simulink model "atrias_gear_dynamics"  (R2017a)
settings: Solver=ode45  StartTime=0.0  StopTime=sim_t  RelTol=1e-3  EnableMultiTasking=on
values from neighbouring files (symbols this model uses):
  N = grid_slice*1000    [createGrid.m]
  nm = fn_set_vnmc_params(sm, sample_time)    [kernel_scores_NM_mismatch.m]    (also in main_ATRIAS_cluster.m)
  nmc_BLCtrlPar = nmc.BLCtrlPar    [kernel_scores_NM_mismatch.m]    (also in main_ATRIAS_cluster.m)
  nmc_FPCtrlPar = nmc.FPCtrlPar    [kernel_scores_NM_mismatch.m]    (also in main_ATRIAS_cluster.m)
  nmc_LLCtrlPar = nmc.LLCtrlPar    [kernel_scores_NM_mismatch.m]    (also in main_ATRIAS_cluster.m)
  nmc_StCtrlPar = nmc.StCtrlPar    [kernel_scores_NM_mismatch.m]    (also in main_ATRIAS_cluster.m)
  nmc_SwCtrlPar = nmc.SwCtrlPar    [kernel_scores_NM_mismatch.m]    (also in main_ATRIAS_cluster.m)
  nmc_TrCtrlPar = nmc.TrCtrlPar    [kernel_scores_NM_mismatch.m]    (also in main_ATRIAS_cluster.m)
  nStep_switchCtrl = 10    [main_ATRIAS_cluster.m]
  nStep_thr = 1000    [createSimInitial.m]    (also in main_ATRIAS_cluster.m)
  rc_CtrlPar = [rc.k_placement, rc.T_step, rc.Cd, rc.kpt, rc.kdt, rc.desired_theta, rc.desired_z, rc.kpz, rc.kdz]    [kernel_scores_NM_mismatch.m]    (also in main_ATRIAS_cluster.m)
  sm = fn_set_MechParams(sm)    [kernel_scores_NM_mismatch.m]    (also in main_ATRIAS_cluster.m = fn_set_MechParams(sm,perturb))
  test_VNMC = 1    [createSimInitial.m]    (also in main_ATRIAS_cluster.m = 0)
undefined symbols (not defined in the file or in its folder): delta_phi_max, delta_phi_max_buffer, delta_phi_min, DiscIntNeverNeededParam, Discrete, idc, initial_dx_estimate, initial_dy_estimate, initial_dz_estimate, initial_z_estimate, kd_shin_max, kd_shin_min, kd_splay_max, kd_splay_min, kd_thigh_max, kd_thigh_min, kp_shin_max, kp_shin_min, kp_splay_max, kp_splay_min, kp_thigh_max, kp_thigh_min, mc, min_splay_angle, min_splay_buffer, phi_shin_max, phi_shin_max_buffer, phi_shin_min, phi_shin_min_buffer, phi_thigh_max, phi_thigh_max_buffer, phi_thigh_min, phi_thigh_min_buffer, rad, rc, s, sample_time, sgn, sim_d, t_friction, Time, X, Y, Z
libraries: sm_lib x206, nesl_utility x132, simulink x77, simulink_extras x24, mblibv1 x4, ctrlSharedLib x4, commnoisgen2 x1, dspswit3 x1
(part 2 of 17)

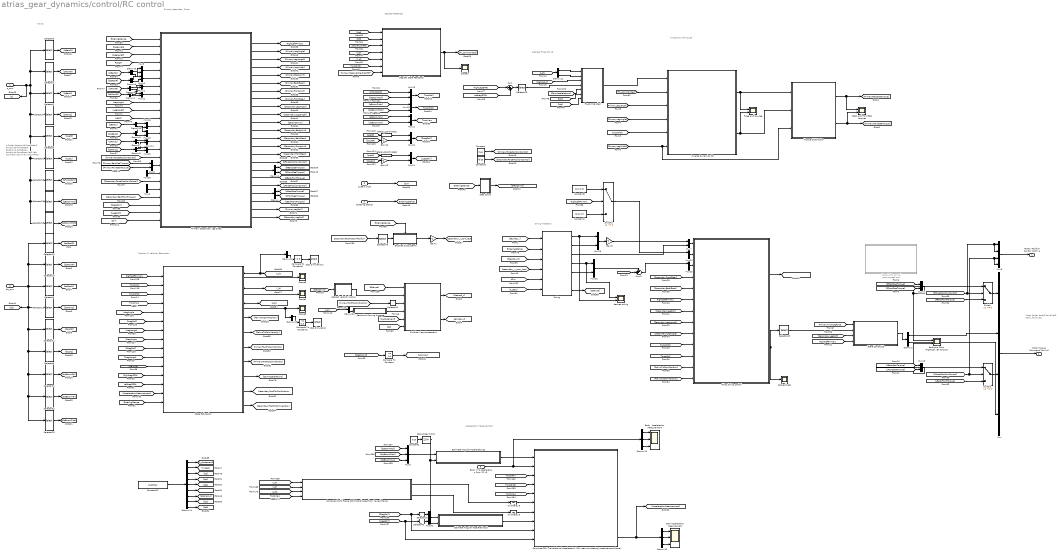
== system atrias_gear_dynamics/control/RC control ==
  note: Motor Order:
      |
      | backR
      | frontR
      | latR
      | backL
      | frontL
      | latL
  note: Inverse Dynamics 2D
  note: Desired Fz sent to ID
  note: Primary/secondary Swap
  note: Sagittal Feedback
  note: Swing Trajectory
  note: Inputs
  note: q Order:
      |
      | backJointR
      | backGearR
      | frontJointR
      | frontGearR
      |
      | backJointL
      | backGearL
      | frontJointL
      | frontGearL
      |
      | latR
      | latL
      |
      | boomRoll
      | boomYaw
      | boomPitch
  note: Position & Velocity Estimation
  note: Acceleration Measurement
  q_cmu : Inport
  dq_cmu : Inport  Port=2
  system clock : Inport  Port=3
  Entering Stance : Inport  Port=4
  Body XYZ Acceleration [m/s^2] x3 : Inport  Port=5
  Atrias Swing control : Subsystem
  Back and Front Right/Left SEA torques : Scope  NumInputPorts=2
  Back and Front SEA torques : Scope  NumInputPorts=2
  Body  Acceleration Measurement : Scope  NumInputPorts=3
  COM Acceleration Measurement : Scope  NumInputPorts=3
  Compare To Constant : simulink/Logic and Bit Operations/Compare To Constant  relop=>=  const=1.0  OutDataTypeStr=boolean
  Compare To Constant1 : simulink/Logic and Bit Operations/Compare To Constant  relop=<=  const=0.3  OutDataTypeStr=boolean
  Compare To Constant2 : simulink/Logic and Bit Operations/Compare To Constant  relop=>=  const=5  OutDataTypeStr=boolean
  Compute COM Translational Acceleration (IMU uses non-rotating measurement frame) : MATLAB Function  TreatAsAtomicUnit=on
  Compute World Frame COM Coordinates from Yawed Frame : MATLAB Function  TreatAsAtomicUnit=on
  Constant : Constant  Value=true
  Constant1 : Constant  Value=false
  Constant12 : Constant  Value=rc_CtrlPar
  Constant2 : Constant  Value=true
  Constant4 : Constant  Value=[0.12 0]
  Constant8 : Constant  Value=[-0.12 0]
  Demux{,1..11,15..16,21} (15 alike) : Demux  Outputs=2
  Demux12 : Demux  Outputs=3
  Demux13 : Demux  Outputs=3
  Demux14 : Demux  Outputs=9
  Enabled Subsystem1 : Subsystem  TreatAsAtomicUnit=on
  Estimate Angular Accelerations2 : Subsystem
  Estimate Angular Accelerations3 : Subsystem
  F_leg and tau_leg : Scope  NumInputPorts=2
  Fz_commanded : Subsystem
  Gain{1,5,12..13} (4 alike) : Gain  Gain=-1
  Inverse Dynamics 2D : Subsystem
  Mux : Mux
  Mux{6..26,28,30,32} (24 alike) : Mux  Inputs=2
  Mux3 : Mux
  Mux5 : Mux  Inputs=3
  Primary Secondary Leg Swap : Subsystem
  Recursive Moving Average : Subsystem
  Sagittal State Feedback : MATLAB Function  TreatAsAtomicUnit=on
  Scope{1,3..5} (4 alike) : Scope
  Selector1 : Selector  InputPortWidth=13  IndexOptions=Index vector (dialog)  Indices=[10]  OutputSizes=1
  Selector10 : Selector  InputPortWidth=13  IndexOptions=Index vector (dialog)  Indices=[7 8]  OutputSizes=1
  Selector11 : Selector  InputPortWidth=13  IndexOptions=Index vector (dialog)  Indices=[9]  OutputSizes=1
  Selector12 : Selector  InputPortWidth=13  IndexOptions=Index vector (dialog)  Indices=[1 2]  OutputSizes=1
  Selector13 : Selector  InputPortWidth=13  IndexOptions=Index vector (dialog)  Indices=[3 4]  OutputSizes=1
  Selector15 : Selector  InputPortWidth=2  IndexOptions=Index vector (dialog)  Indices=[2]  OutputSizes=1
  Selector16 : Selector  InputPortWidth=2  IndexOptions=Index vector (dialog)  Indices=[2]  OutputSizes=1
  Selector18 : Selector  InputPortWidth=13  IndexOptions=Index vector (dialog)  Indices=[13]  OutputSizes=1
  Selector2 : Selector  InputPortWidth=13  IndexOptions=Index vector (dialog)  Indices=[5 6]  OutputSizes=1
  Selector20 : Selector  InputPortWidth=13  IndexOptions=Index vector (dialog)  Indices=[13]  OutputSizes=1
  Selector21 : Selector  InputPortWidth=13  IndexOptions=Index vector (dialog)  Indices=[11]  OutputSizes=1
  Selector22 : Selector  InputPortWidth=13  IndexOptions=Index vector (dialog)  Indices=[12]  OutputSizes=1
  Selector23 : Selector  InputPortWidth=13  IndexOptions=Index vector (dialog)  Indices=[11]  OutputSizes=1
  Selector28 : Selector  InputPortWidth=13  IndexOptions=Index vector (dialog)  Indices=[12]  OutputSizes=1
  Selector4 : Selector  InputPortWidth=13  IndexOptions=Index vector (dialog)  Indices=[7 8]  OutputSizes=1
  Selector40 : Selector  InputPortWidth=3  IndexOptions=Index vector (dialog)  Indices=[1 2]  OutputSizes=1
  Selector41 : Selector  InputPortWidth=3  IndexOptions=Index vector (dialog)  Indices=1  OutputSizes=1
  Selector42 : Selector  InputPortWidth=2  IndexOptions=Index vector (dialog)  Indices=[2]  OutputSizes=1
  Selector43 : Selector  InputPortWidth=3  IndexOptions=Index vector (dialog)  Indices=[1]  OutputSizes=1
  Selector5 : Selector  InputPortWidth=13  IndexOptions=Index vector (dialog)  Indices=[9]  OutputSizes=1
  Selector6 : Selector  InputPortWidth=13  IndexOptions=Index vector (dialog)  Indices=[1 2]  OutputSizes=1
  Selector7 : Selector  InputPortWidth=13  IndexOptions=Index vector (dialog)  Indices=[3 4]  OutputSizes=1
  Selector8 : Selector  InputPortWidth=13  IndexOptions=Index vector (dialog)  Indices=[10]  OutputSizes=1
  Selector9 : Selector  InputPortWidth=13  IndexOptions=Index vector (dialog)  Indices=[5 6]  OutputSizes=1
  Simbicon leg placcement : Subsystem
  State Estimation : Subsystem
  Step Count : Subsystem
  Stop Simulation : Stop
  Stop Simulation1 : Stop
  Sum : Sum  Inputs=|++
  Sum2 : Sum  Inputs=-+|
  Swing : Subsystem
  Switch : Switch  Criteria=u2 ~= 0
  Switch1 : Switch  Criteria=u2 ~= 0
  Switch2 : Switch  Criteria=u2 ~= 0
  Torque Distribution : Subsystem
  Unit Delay5 : UnitDelay  SampleTime=sample_time
  Unit Delay6 : UnitDelay  SampleTime=sample_time
  Zero-Order Hold1 : ZeroOrderHold  SampleTime=sample_time
  desired beta : Scope
  desired swing : Scope  NumInputPorts=2
  desired velocity lookup : MATLAB Function  TreatAsAtomicUnit=on
  lateralControl2D : Subsystem
  lateral_PID_control : Subsystem  Commented=on
  lateral_coordinates : Fcn  Expr=pi/2-u
  lateral_coordinates1 : Fcn  Expr=pi/2-u
  Force / Position Control [1/0] x4 : Outport  OutputWhenDisabled=reset  InitialOutput=[0 0 0 0 0 0]
  Motor Torque Command [Nm] x6 : Outport  Port=2  OutputWhenDisabled=reset  InitialOutput=[0 0 0 0 0 0]
  tag scope: EnteringStance=global, PrimaryFootToComPosition=global, RightLeftPrimary=global, SecondaryFootToComPosition=global, TorsoPitch=global, TorsoRoll=global, TorsoYaw=global, X_dX=global, Y_dY=global, Z_dZ=global, desired_xd=global, tSim=global
  wires:
  ? -> Mux20/2
  [LLegRoll] -> State Estimation/6(Left Leg Roll [rad rad/s])
  Selector9/1 -> [dqBackL]
  ? -> Mux6/2
  ? -> Mux26/2
  ? -> Mux6/1
  desired velocity lookup/1(desired_xd) -> Simbicon leg placcement/2(dx_des [m/s])
  State Estimation/7(Primary Foot to COM Velocity [m/s m/s m/s]) -> [PrimaryFootToComVelocity]
  State Estimation/6(Primary Foot to COM Position [m m m]) -> [PrimaryFootToComPosition]
  State Estimation/1("Horizontal COM [m, m/s]") -> Scope3/1, Demux16/1, [X_dX]
  Selector1/1 -> [qLatL]
  Selector2/1 -> [qBackL]
  ? -> Mux26/1
  Selector7/1 -> [qFrontR]
  Selector6/1 -> [qBackR]
  ? -> Mux25/2
  Selector12/1 -> [dqBackR]
  Selector11/1 -> [dqLatR]
  Selector8/1 -> [dqLatL]
  Selector22/1 -> [dqBoomYaw]
  [RLegLength] -> State Estimation/10(Right Leg Length [m m/s])
  [LLegAngle] -> State Estimation/5(Left Leg Sagittal Angle [rad rad/s])
  [TorsoPitch] -> State Estimation/3(Torso Pitch [rad rad/s])
  dq_cmu/1 -> Selector9/1, Selector13/1, Selector12/1, [dq], Selector10/1, Selector11/1, Selector8/1, Selector21/1, Selector22/1, Selector20/1
  Selector13/1 -> [dqFrontR]
  State Estimation/10(Secondary to COM Velocity [m/s m/s m/s]) -> [SecondaryFootToComVelocity]
  Selector21/1 -> [dqBoomRoll]
  Selector20/1 -> [dqBoomPitch]
  [RLegRoll] -> State Estimation/9(Right Leg Roll [rad rad/s])
  Selector23/1 -> [qTorsoRoll]
  Selector18/1 -> [qBoomPitch]
  [TorsoRoll] -> State Estimation/2(Torso Roll [rad rad/s])
  Selector28/1 -> [qBoomYaw]
  Selector4/1 -> [qFrontL]
  q_cmu/1 -> [q], Selector1/1, Selector23/1, Selector28/1, Selector18/1, Selector5/1, Selector4/1, Selector2/1, Selector7/1, Selector6/1
  Selector10/1 -> [dqFrontL]
  Demux21/2 -> Recursive Moving Average/1(dx [m/s])
  Gain1/1 -> [secondary_x_com_last]
  State Estimation/4(Pelvis to COM Position [m m m]) -> [PelvisToComPosition]
  [LLegLength] -> State Estimation/7(Left Leg Length [m m/s])
  State Estimation/9(Secondary to COM Position [m m m]) -> [SecondaryFootToComPosition]
  [tStance] -> Simbicon leg placcement/1(Ts [s])
  Selector5/1 -> [qLatR]
  Entering Stance/1 -> [EnteringStance]
  [desired_x] -> Swing/1(desired_x)
  Simbicon leg placcement/1(desired_footsstep) -> [desired_x]
  [TorsoYaw] -> State Estimation/4(Torso Yaw [rad rad/s])
  [PrimaryFootToComPosition] -> Selector41/1
  [X_dX] -> Demux21/1
  [PrimaryLegLength] -> Inverse Dynamics 2D/3(Leg Length [m m/s])  "Primary Leg Length [position, velocity]"
  [PrimaryLegAngle] -> Inverse Dynamics 2D/4(Leg Angle [rad rad/s])  "Primary Leg Angle  [position, velocity]"
  [TorsoPitch] -> Inverse Dynamics 2D/5(Torso Pitch [rad rad/s])  "Torso Pitch [position, velocity]"
  [PrimaryLegWidth] -> Inverse Dynamics 2D/6(Primary w [m]), Torque Distribution/3(Primary Leg Width [m])
  Inverse Dynamics 2D/1(Leg Force [N]) -> F_leg and tau_leg/1, Torque Distribution/1(Leg Force [N])  "Virtual Leg Force to Command"
  Inverse Dynamics 2D/2(Leg Torque [Nm]) -> F_leg and tau_leg/2, Torque Distribution/2(Leg Torque [Nm])  "Virtual Leg Torque to Command"
  Torque Distribution/1(Back Torque [Nm]) -> Back and Front SEA torques/1, [PrimaryBackSeaTorque]
  Torque Distribution/2(Front Torque [Nm]) -> Back and Front SEA torques/2, [PrimaryFrontSeaTorque]
  [SecondaryBackFrontTorque] -> Primary Secondary Leg Swap/21(Secondary Back/Front Motor Torque [Nm Nm])
  Mux26/1 -> Primary Secondary Leg Swap/18(Primary Back/Front Motor Torque [Nm Nm])
  [SecondaryForcePositionControl] -> Primary Secondary Leg Swap/19(Secondary Force/Position Control [1/0])
  [PrimaryForcePositionControl] -> Primary Secondary Leg Swap/16(Primary Force/Position Control [1/0])
  Demux9/2 -> Mux13/2
  Demux9/1 -> Mux16/2
  Demux10/2 -> Mux13/1
  Demux10/1 -> Mux16/1
  [qBackL] -> Demux10/1
  [dqBackL] -> Demux9/1
  Demux8/2 -> Mux15/2
  Demux8/1 -> Mux14/2
  Demux7/2 -> Mux15/1
  Demux7/1 -> Mux14/1
  Mux15/1 -> Primary Secondary Leg Swap/15(L Front Gear [rad rad/s])
  Mux14/1 -> Primary Secondary Leg Swap/14(L Front Joint [rad rad/s])
  Mux13/1 -> Primary Secondary Leg Swap/13(L Back Gear [rad rad/s])
  Mux16/1 -> Primary Secondary Leg Swap/12(L Back Joint [rad rad/s])
  [dqFrontL] -> Demux8/1
  [qFrontL] -> Demux7/1
  Demux5/2 -> Mux10/2
  Demux5/1 -> Mux9/2
  Demux6/2 -> Mux10/1
  Demux6/1 -> Mux9/1
  [qBackR] -> Demux6/1
  [dqBackR] -> Demux5/1
  Demux4/2 -> Mux12/2
  Demux4/1 -> Mux11/2
  Demux3/2 -> Mux12/1
  Demux3/1 -> Mux11/1
  Mux12/1 -> Primary Secondary Leg Swap/8(R Front Gear [rad rad/s])
  Mux11/1 -> Primary Secondary Leg Swap/7(R Front Joint [rad rad/s])
  Mux10/1 -> Primary Secondary Leg Swap/6(R Back Gear [rad rad/s])
  Mux9/1 -> Primary Secondary Leg Swap/5(R Back Joint [rad rad/s])
  [dqFrontR] -> Demux4/1
  [qFrontR] -> Demux3/1
  [PrimaryBackSeaTorque] -> Mux8/1
  [PrimaryFrontSeaTorque] -> Mux8/2
  Mux8/1 -> Primary Secondary Leg Swap/17(Primary Back/Front SEA Torque [Nm Nm])
  Mux6/1 -> Primary Secondary Leg Swap/20(Secondary Back/Front SEA Torque [Nm Nm])
  [LLegW] -> Primary Secondary Leg Swap/11(L Leg w [m])
  [LLegLength] -> Primary Secondary Leg Swap/10(L Leg Length [m m/s])
  [LLegAngle] -> Primary Secondary Leg Swap/9(L Leg Angle [rad rad/s])
  [RLegW] -> Primary Secondary Leg Swap/4(R Leg w [m])
  [RLegLength] -> Primary Secondary Leg Swap/3(R Leg Length [m m/s])
  [RLegAngle] -> Primary Secondary Leg Swap/2(R Leg Angle [rad rad/s])
  [RLegRoll] -> Primary Secondary Leg Swap/22("Right Leg Roll [rad, rad/s]")
  [LLegRoll] -> Primary Secondary Leg Swap/23("Left Leg Roll [rad, rad/s]")
  Primary Secondary Leg Swap/1(Right/Left Primary [1/0]) -> [RightLeftPrimary]
  Primary Secondary Leg Swap/21(L Back/Front Motor Torque [Nm Nm]) -> [LBackFrontTorque]
  Primary Secondary Leg Swap/18(R Back/Front Motor Torque [Nm Nm]) -> [RBackFrontTorque]
  Primary Secondary Leg Swap/16(R Force/Position Control [1/0]) -> [RForcePositionControl]
  Primary Secondary Leg Swap/19(L Force/Position Control [1/0]) -> [LForcePositionControl]
  Primary Secondary Leg Swap/11(Secondary Leg w [m]) -> [SecondaryW]
  Primary Secondary Leg Swap/15(Secondary Front Gear [rad rad/s]) -> [SecondaryFrontGear]
  Primary Secondary Leg Swap/14(Secondary Front Joint [rad rad/s]) -> [SecondaryFrontJoint]
  Primary Secondary Leg Swap/13(Secondary Back Gear [rad rad/s]) -> [SecondaryBackGear]
  Primary Secondary Leg Swap/12(Secondary Back Joint [rad rad/s]) -> [SecondaryBackJoint]
  Primary Secondary Leg Swap/8(Primary Front Gear [rad rad/s]) -> [PrimaryFrontGear]
  Primary Secondary Leg Swap/7(Primary Front Joint [rad rad/s]) -> [PrimaryFrontJoint]
  Primary Secondary Leg Swap/6(Primary Back Gear [rad rad/s]) -> [PrimaryBackGear]
  Primary Secondary Leg Swap/5(Primary Back Joint [rad rad/s]) -> [PrimaryBackJoint]
  Demux1/2 -> [RFrontSeaTorque]
  Demux1/1 -> [RBackSeaTorque]
  Primary Secondary Leg Swap/17(R Back/Front SEA Torque [Nm Nm]) -> Demux1/1
  Demux/2 -> [LFrontSeaTorque]
  Demux/1 -> [LBackSeaTorque]
  Primary Secondary Leg Swap/20(L Back/Front SEA Torque [Nm Nm]) -> Demux/1
  Primary Secondary Leg Swap/9(Secondary Leg Angle [rad rad/s]) -> [SecondaryLegAngle]
  Primary Secondary Leg Swap/10(Secondary Leg Length [rad rad/s]) -> [SecondaryLegLength]
  Primary Secondary Leg Swap/3(Primary Leg Length [m m/s]) -> [PrimaryLegLength]
  Primary Secondary Leg Swap/4(Primary Leg w [m]) -> [PrimaryLegWidth]
  Primary Secondary Leg Swap/2(Primary Leg Angle [rad rad/s]) -> [PrimaryLegAngle]
  Primary Secondary Leg Swap/22("Primary Leg Roll [rad, rad/s]") -> [PrimaryLegRoll]
  Primary Secondary Leg Swap/23("Secondary Leg Roll [rad, rad/s]") -> [SecondaryLegRoll]
  Switch1/1 -> Mux/3
  [LBackFrontTorque] -> Switch1/3
  [RBackFrontTorque] -> Switch/3
  Demux2/1 -> Mux/2
  Switch/1 -> Mux/1
  [LForcePositionControl] -> Switch1/2, Mux3/3, Mux3/4
  [RForcePositionControl] -> Switch/2, Mux3/1, Mux3/2
  Mux3/1 -> Force / Position Control [1/0] x4/1
  Mux/1 -> Motor Torque Command [Nm] x6/1
  Demux2/2 -> Mux/4
  [RBackSeaTorque] -> Mux17/1
  [RFrontSeaTorque] -> Mux17/2
  Mux17/1 -> Switch/1, Back and Front Right/Left SEA torques/1
  [LBackSeaTorque] -> Mux18/1
  [LFrontSeaTorque] -> Mux18/2
  Mux18/1 -> Back and Front Right/Left SEA torques/2, Switch1/1
  Constant/1 -> [PrimaryForcePositionControl]
  Constant1/1 -> [SecondaryForcePositionControl]
  [SecondaryFrontGear] -> Atrias Swing control/4(Secondary Front Gear [rad rad/s])
  [SecondaryBackGear] -> Atrias Swing control/5(Secondary Back Gear [rad rad/s])
  [dqBoomYaw] -> Mux21/2
  [qBoomYaw] -> Mux21/1
  [qBoomPitch] -> Mux19/1
  Gain12/1 -> Mux22/2
  Gain13/1 -> Mux24/2
  lateral_coordinates1/1 -> Mux24/1
  lateral_coordinates/1 -> Mux22/1
  Mux24/1 -> [LLegRoll]
  Mux22/1 -> [RLegRoll]
  [dqLatL] -> Gain13/1
  [qLatL] -> lateral_coordinates1/1
  [dqLatR] -> Gain12/1
  [qLatR] -> lateral_coordinates/1
  [dqBoomPitch] -> Mux19/2
  Mux19/1 -> [TorsoPitch]
  Mux23/1 -> [TorsoRoll]
  Mux21/1 -> [TorsoYaw]
  [dqBoomRoll] -> Mux23/2
  [qTorsoRoll] -> Mux23/1
  Atrias Swing control/1(Back Front Motor Torques [Nm Nm]) -> [SecondaryBackFrontTorque]
  Atrias Swing control/2(Desired Swing Beta [rad rad/s]) -> Selector40/1, desired beta/1
  [RightLeftPrimary] -> Atrias Swing control/6(Right or Left Stance [1 or 0])
  [SecondaryLegRoll] -> Atrias Swing control/7(Secondary Leg Roll [rad rad/s])
  [TorsoRoll] -> Atrias Swing control/11(Torso Roll [rad rad/s])
  [TorsoPitch] -> Atrias Swing control/10(Torso Pitch [rad rad/s])
  [SecondaryLegAngle] -> Atrias Swing control/9(Secondary Leg Angle [rad rad/s])
  [SecondaryLegLength] -> Atrias Swing control/8(Secondary Leg Length [m m/s])
  Sum2/1 -> Mux25/1
  [Z_dZ] -> Sum2/2
  Mux20/1 -> Atrias Swing control/2(Y COM  from Secondary Foot Desired [m m/s m/s^2])
  Mux25/1 -> Atrias Swing control/3(Z COM  from Secondary Foot Desired [m m/s m/s^2])
  [RightLeftPrimary] -> lateralControl2D/4(RightLeftPrimary [1 or 0])
  [Z_dZ] -> Demux11/1
  Demux11/1 -> Fz_commanded/1(measured_z)
  [TorsoPitch] -> Sagittal State Feedback/6(theta_dtheta)
  [Z_dZ] -> Sagittal State Feedback/5(z_dz)
  Mux7/1 -> Atrias Swing control/1(X COM from Secondary Foot Desired [m m/s m/s^2])
  Mux32/1 -> Sum2/1
  [PelvisToComPosition] -> Atrias Swing control/12(Pelvis to COM Position [m] x3)
  [PelvisToComVelocity] -> Atrias Swing control/13(Pelvis to COM Velocity [m/s] x3)
  [EnteringStance] -> Primary Secondary Leg Swap/1(Entering Stance [1/0])
  [RightLeftPrimary] -> Switch2/2
  Switch2/1 -> Mux20/1
  Constant8/1 -> Switch2/1
  Constant4/1 -> Switch2/3
  [X_dX] -> Sagittal State Feedback/4(x_dx)
  [tSim] -> Primary Secondary Leg Swap/24(System Time [s])
  [EnteringStance] -> Step Count/1(In1)
  Step Count/1(Out1) -> [StepCount]
  [PrimaryMeasuredVerticalGRF] -> Sagittal State Feedback/7(GRF_z)
  Demux11/2 -> Fz_commanded/2(measured_zd)
  Fz_commanded/1(Fz_commanded) -> Inverse Dynamics 2D/1(Desired Vertical GRF [N])
  Sagittal State Feedback/1(Fx) -> [Fx_commanded], Scope1/1
  [Fx_commanded] -> Inverse Dynamics 2D/2(Desired Forward GRF [N])
  [EnteringStance] -> Swing/2(EnteringStance)
  [StepCount] -> Swing/3(nstep)
  [tSim] -> Swing/5(tSim)
  Swing/2(xd) -> Mux28/2
  Swing/5(zd) -> Mux32/2
  Swing/7(tStance_last) -> [tStance]
  Swing/1(x) -> desired swing/2, Mux28/1
  Swing/4(z) -> desired swing/1, Mux32/1
  lateralControl2D/1(Lateral Torque command [R L]) -> Demux2/1
  Swing/3(xdd) -> Mux7/2
  [secondary_x_com_last] -> Swing/4(secondary_x)
  Mux28/1 -> Gain5/1
  Gain5/1 -> Mux7/1
  Enabled Subsystem1/1(Out1) -> Gain1/1
  [EnteringStance] -> Enabled Subsystem1/Enable
  [SecondaryFootToComPosition] -> Selector43/1
  Selector43/1 -> Enabled Subsystem1/1(In1)
  Selector41/1 -> Simbicon leg placcement/3(Foot2CoM)
  system clock/1 -> [tSim]
  State Estimation/2("Lateral COM [m, m/s]") -> Scope4/1, [Y_dY]
  State Estimation/5(Pelvis to COM Velocity [m/s m/s m/s]) -> [PelvisToComVelocity]
  [RightLeftPrimary] -> State Estimation/1(Right or Left [1/0])
  Recursive Moving Average/1(dx_avg [m/s]) -> Simbicon leg placcement/4(dx_avg [m/s])
  [RLegAngle] -> State Estimation/8(Right Leg Sagittal Angle [rad rad/s])
  [RightLegGRFs] -> State Estimation/12(Right GRF [X Z] [N N])
  [LeftLegGRFs] -> State Estimation/13(Left GRF [X Z] [N N])
  [EnteringStance] -> State Estimation/15(Entering Stance [1/0])
  [AccelerationMeasurement] -> State Estimation/14(" Acceleration Measurement [m/s^2] x3")
  [TorsoYaw] -> Compute World Frame COM Coordinates from Yawed Frame/4(torso_yaw)
  [Z_dZ] -> Compute World Frame COM Coordinates from Yawed Frame/3(Z_dZ)
  [Y_dY] -> Compute World Frame COM Coordinates from Yawed Frame/2(Y_dY)
  [X_dX] -> Compute World Frame COM Coordinates from Yawed Frame/1(X_dX)
  Compute World Frame COM Coordinates from Yawed Frame/1(com_position_world) -> Unit Delay5/1
  Compute World Frame COM Coordinates from Yawed Frame/2(com_velocity_world) -> Unit Delay6/1
  Unit Delay6/1 -> Compute COM Translational Acceleration (IMU uses non-rotating measurement frame)/7(com_velocity_world)
  Unit Delay5/1 -> Compute COM Translational Acceleration (IMU uses non-rotating measurement frame)/6(com_position_world)
  [TorsoYaw] -> Compute COM Translational Acceleration (IMU uses non-rotating measurement frame)/5(torso_yaw)
  Estimate Angular Accelerations3/1(Angular Accelerations [rad/s^2] x2) -> Compute COM Translational Acceleration (IMU uses non-rotating measurement frame)/8(hip_roll_accelerations)
  Estimate Angular Accelerations2/1(Angular Accelerations [rad/s^2] x3) -> Compute COM Translational Acceleration (IMU uses non-rotating measurement frame)/1(torso_angular_accelerations)
  Zero-Order Hold1/1 -> Estimate Angular Accelerations3/2(Enabled), Estimate Angular Accelerations2/2(Enabled)
  Mux5/1 -> Estimate Angular Accelerations2/1(Angular Velocities [rad/s] x3)
  [TorsoRoll] -> Compute COM Translational Acceleration (IMU uses non-rotating measurement frame)/3(torso_roll)
  [TorsoPitch] -> Compute COM Translational Acceleration (IMU uses non-rotating measurement frame)/4(torso_pitch)
  Demux12/3 -> COM Acceleration Measurement/3
  Demux12/1 -> COM Acceleration Measurement/1
  Demux12/2 -> COM Acceleration Measurement/2
  Compute COM Translational Acceleration (IMU uses non-rotating measurement frame)/6(com_acceleration_yawed) -> [AccelerationMeasurement], Demux12/1
  [dqBoomRoll] -> Mux5/1
  [dqBoomPitch] -> Mux5/2
  [dqBoomYaw] -> Mux5/3
  Mux30/1 -> Estimate Angular Accelerations3/1(Angular Velocities [rad/s] x2)
  Selector42/1 -> Mux30/2
  Selector16/1 -> Mux30/1
  [LLegRoll] -> Compute COM Translational Acceleration (IMU uses non-rotating measurement frame)/10(left_hip_roll), Selector42/1
  [RLegRoll] -> Compute COM Translational Acceleration (IMU uses non-rotating measurement frame)/9(right_hip_roll), Selector16/1
  [walking] -> State Estimation/11(Enable Kalman Filtering [1/0])
  [StepCount] -> Compare To Constant/1
  Compare To Constant/1 -> [walking]
  Constant2/1 -> Zero-Order Hold1/1
  State Estimation/8(COM Acceleration [m/s^2] x3) -> [ComAccelerations]
  [ComAccelerations] -> Fz_commanded/5(COM XYZ Acceleration [m/s^2] x3)
  [SecondaryLegRoll] -> lateralControl2D/3(SecondaryLegRoll)
  Selector40/1 -> lateralControl2D/2(desired_SecondaryLegRoll)
  [PrimaryAxialLegForce] -> lateralControl2D/1(Primary Axial Leg Force [N])
  Demux13/3 -> Body  Acceleration Measurement/3
  Demux13/1 -> Body  Acceleration Measurement/1
  Demux13/2 -> Body  Acceleration Measurement/2
  Body XYZ Acceleration [m/s^2] x3/1 -> Demux13/1, Compute COM Translational Acceleration (IMU uses non-rotating measurement frame)/2(imu_translational_accelerations_body)
  [k_placement] -> Simbicon leg placcement/5(k_placement)
  [T_step] -> Swing/6(T_step)
  [Cd] -> Simbicon leg placcement/6(Cd)
  [kpt] -> Sagittal State Feedback/1(kpt)
  [kdt] -> Sagittal State Feedback/2(kdt)
  Selector15/1 -> Fz_commanded/4("Primary Measured Vertical [N}")
  State Estimation/3("Vertical COM [m, m/s]") -> Demux15/1, Scope5/1, [Z_dZ]
  Compare To Constant1/1 -> Stop Simulation/1
  Demux15/1 -> Compare To Constant1/1
  Compare To Constant2/1 -> Stop Simulation1/1
  Demux16/2 -> Compare To Constant2/1
  [StepCount] -> desired velocity lookup/1(nStep)
  [RightLegGRFs] -> Sum/1
  [LeftLegGRFs] -> Sum/2
  Sum/1 -> Selector15/1
  Simbicon leg placcement/2(desired_speed) -> [desired_xd]
  [desired_theta] -> Sagittal State Feedback/3(desired_theta)
  [desired_z] -> Fz_commanded/3(desired_z)
  [kpz] -> Fz_commanded/6(kpz)
  [kdz] -> Fz_commanded/7(kdz)
  Demux14/9 -> [kdz]
  Demux14/2 -> [T_step]
  Demux14/5 -> [kdt]
  Demux14/4 -> [kpt]
  Constant12/1 -> Demux14/1
  Demux14/6 -> [desired_theta]
  Demux14/8 -> [kpz]
  Demux14/7 -> [desired_z]
  Demux14/3 -> [Cd]
  Demux14/1 -> [k_placement]

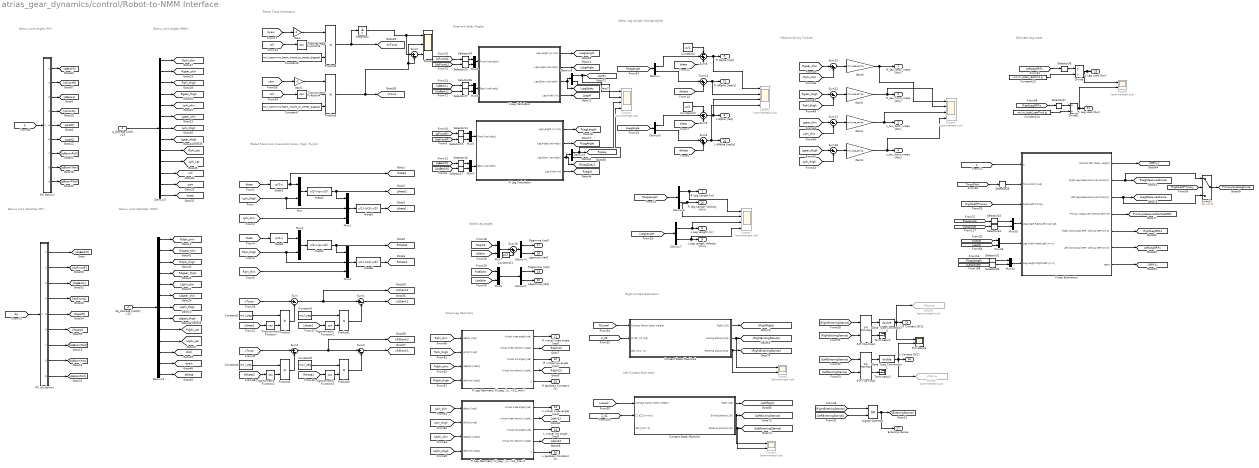
== system atrias_gear_dynamics/control/Robot-to-NMM Interface ==
  note: Global Robot Link Kinematics
      | (torso, thigh, fb_link)
  note: Planar Torso Kinematics
  note: Alpha, Leg Length
      | (change alpha)
  note: Demux Joint
      | Angles (NMC)
  note: Demux Joint
      | Velocities (NMC)
  note: Knee and Splay Angles
  note: Virtual Leg Geometry
  note: Measure Spring Torques
  note: Estimate Leg Loads
  note: Global Leg Angles
  note: Demux Joint
      | Angles (RC)
  note: Demux Joint
      | Velocities (RC)
  note: Left Contact Estimation
  note: Right Contact Estimation
  q_discrete [rad] x13 : Inport
  dq_discrete [rad/2] x13 : Inport  Port=2
  Constant1 : Constant  Value=pi/2
  Constant11 : Constant  Value=pi/2
  Constant12 : Constant  Value=pi/2
  Constant13 : Constant  Value=mc.m_total_real*mc.g
  Constant14 : Constant  Value=mc.m_total_real*mc.g
  Constant{2..5} (4 alike) : Constant  Value=mc.l_seg
  Constant6 : Constant  Value=mc.l_boom+mc.boom_mount_to_center_diagonal
  Constant7 : Constant  Value=mc.l_boom+mc.boom_mount_to_center_diagonal
  Contact State Machine : Subsystem
  Contact State Machine1 : Subsystem
  Data Type Conversion1 : DataTypeConversion  OutDataTypeStr=double
  Data Type Conversion3 : DataTypeConversion  OutDataTypeStr=double
  Demux{,1,4..9} (8 alike) : Demux  Outputs=2
  Demux2 : Demux  Outputs=13
  Demux3 : Demux  Outputs=13
  Divide : Product  Inputs=*/
  Divide1 : Product  Inputs=*/
  Force Estimation : Subsystem
  Gain : Gain  Gain=-1
  Gain1 : Gain  Gain=-1
  Gain{3..6} (4 alike) : Gain  Gain=mc.k_leg_spring
  Goto81 : Goto  Commented=on  GotoTag=RStance  TagVisibility=global
  Goto84 : Goto  Commented=on  GotoTag=LStance  TagVisibility=global
  Integrator : Integrator
  L Leg Calculator : Subsystem
  Logical Operator : Logic  Operator=OR  AllPortsSameDT=off  OutDataTypeStr=boolean
  Mux{,2,4..9,33..35} (11 alike) : Mux  Inputs=2
  Mux1 : Mux  Inputs=3
  Mux3 : Mux  Inputs=3
  Product{,1..3} (4 alike) : Product
  Product4 : Product  Inputs=3
  Product5 : Product  Inputs=3
  R Leg Calculator : Subsystem
  "R Leg Geometry f(l_seg, l_v, v12_max)" : Subsystem
  "R Leg Geometry f(l_seg, l_v, v12_max)1" : Subsystem
  R/L Stance : Scope  NumInputPorts=2
  RC Demux : Subsystem
  RC dq demux : Subsystem
  S-R Flip-Flop1 : simulink_extras/Flip Flops/S-R Flip-Flop  initial_condition=0
  S-R Flip-Flop2 : simulink_extras/Flip Flops/S-R Flip-Flop  initial_condition=0
  Scope : Scope  NumInputPorts=3
  Scope2 : Scope  Commented=on  NumInputPorts=2
  Scope3 : Scope  Commented=on  NumInputPorts=2
  Scope{4..7} (4 alike) : Scope  Commented=on  NumInputPorts=4
  Scope8 : Scope  Commented=on  NumInputPorts=2
  Selector{14..17,24..27,31..35} (13 alike) : Selector  InputPortWidth=2  IndexOptions=Index vector (dialog)  Indices=[1]  OutputSizes=1
  Selector36 : Selector  InputPortWidth=2  IndexOptions=Index vector (dialog)  Indices=[2]  OutputSizes=1
  Selector37 : Selector  InputPortWidth=2  IndexOptions=Index vector (dialog)  Indices=[2]  OutputSizes=1
  Sum{,1..3,7,10..13} (9 alike) : Sum  Inputs=|+-
  Sum14 : Sum  Inputs=|++
  Sum18 : Sum  Inputs=|++
  Sum4 : Sum  Inputs=|++
  Sum5 : Sum  Inputs=-++
  Sum6 : Sum  Inputs=-++
  Switch1 : Switch  Criteria=u2 ~= 0
  Terminator1 : Terminator
  Terminator2 : Terminator
  Trigonometric Function{,1..4,6} (6 alike) : Trigonometry  Operator=cos
  theta1 : Fcn  Expr=u(1)+(pi-u(2))
  theta2 : Fcn  Expr=u(1)+(pi-u(2))
  theta3 : Fcn  Expr=pi/2-u
  theta4 : Fcn  Expr=pi/2-u
  theta5 : Fcn  Expr=u(1)-(u(3)-u(2))
  theta6 : Fcn  Expr=u(1)-(u(3)-u(2))
  R_tau_back_meas [Nm] : Outport
  R_tau_front_meas [Nm] : Outport  Port=2
  L_tau_back_meas [Nm] : Outport  Port=3
  L_tau_front_meas [Nm] : Outport  Port=4
  R Alpha [rad] : Outport  Port=5
  L Alpha [rad] : Outport  Port=6
  R Leg Length [m] : Outport  Port=7
  L Leg Length [m] : Outport  Port=8
  L Leg Length Velocity [m/s] : Outport  Port=9
  R Leg Length Velocity [m/s] : Outport  Port=10
  R virtual knee angle [rad] : Outport  Port=11
  R virtual hip angle [rad] : Outport  Port=12
  L virtual knee angle [rad] : Outport  Port=13
  L virtual hip angle [rad] : Outport  Port=14
  R Jacobian Constant (k) : Outport  Port=15
  L Jacobian Constant (k) : Outport  Port=16
  Rgamma [rad] : Outport  Port=17
  Lgamma [rad] : Outport  Port=18
  Rdgamma [rad] : Outport  Port=19
  Ldgamma [rad] : Outport  Port=20
  R dAlpha [rad/s] : Outport  Port=21
  L dAlpha [rad/s] : Outport  Port=22
  L Leg Load [bw] : Outport  Port=23
  R Leg Load [bw] : Outport  Port=24
  R Contact [0/1] : Outport  Port=25
  L Contact [0/1] : Outport  Port=26
  Entering stance : Outport  Port=27
  tag scope: LLegAngle=global, LLegLength=global, LLegMeasuredForce=global, LLegSplay=global, LLegW=global, Ldgear_shin=global, Ldgear_thigh=global, Ldphi12=global, Ldphi23=global, Ldphi_Lat=global, Ldphi_shin=global, Ldphi_thigh=global, LeftLegGRFs=global, Lgear_shin=global, Lgear_thigh=global, Lphi_Lat=global, Lphi_shin=global, Lphi_thigh=global, Lsplay=global, Ltheta1=global, Ltheta2=global, PrimaryAxialLegForce=global, PrimaryMeasuredVerticalGRF=global, RLegAngle=global, RLegLength=global, RLegMeasuredForce=global, RLegW=global, Rdgear_shin=global, Rdgear_thigh=global, Rdphi12=global, Rdphi23=global, Rdphi_Lat=global, Rdphi_shin=global, Rdphi_thigh=global, Rgear_shin=global, Rgear_thigh=global, RightLegGRFs=global, Rphi_Lat=global, Rphi_shin=global, Rphi_thigh=global, Rsplay=global, Rtheta1=global, Rtheta2=global, droll=global, dtheta=global, dxTorso=global, dyaw=global, roll=global, theta3=global, theta=global, xLShank1=global, xLShank2=global, xRShank1=global, xRShank2=global, xTorso=global, yaw=global
  wires:
  Sum3/1 -> [xRShank1]
  Sum2/1 -> [xRShank2], Sum3/1
  Product3/1 -> Sum3/2
  Trigonometric Function3/1 -> Product3/2
  Constant2/1 -> Product/1
  Trigonometric Function/1 -> Product/2
  Sum1/1 -> [xLShank1]
  Constant3/1 -> Product1/1
  Trigonometric Function2/1 -> Product2/2
  Product1/1 -> Sum1/2
  [Rtheta2] -> Trigonometric Function2/1
  Sum/1 -> [xLShank2], Sum1/1
  [Ltheta1] -> Trigonometric Function1/1
  Product/1 -> Sum/2
  Product2/1 -> Sum2/2
  [xTorso] -> Sum2/1
  [Rtheta1] -> Trigonometric Function3/1
  Constant4/1 -> Product2/1
  Constant5/1 -> Product3/1
  [xTorso] -> Sum/1
  [Ltheta2] -> Trigonometric Function/1
  Product4/1 -> [dxTorso], Integrator/1
  Trigonometric Function1/1 -> Product1/2
  [dyaw] -> Gain/1
  [theta] -> theta3/1
  [Lphi_thigh] -> Mux1/2, Mux/2
  theta3/1 -> Mux/1, [theta3]
  Mux/1 -> theta2/1
  theta2/1 -> Mux1/1, [Ltheta2]
  Mux1/1 -> theta5/1
  [Lphi_shin] -> Mux1/3
  [theta] -> theta4/1
  [Rphi_thigh] -> Mux3/2, Mux2/2
  theta4/1 -> Mux2/1
  Mux2/1 -> theta1/1
  theta1/1 -> Mux3/1, [Rtheta2]
  Mux3/1 -> theta6/1
  [Rphi_shin] -> Mux3/3
  theta5/1 -> [Ltheta1]
  theta6/1 -> [Rtheta1]
  [theta] -> Sum6/3
  Constant1/1 -> Sum6/1
  Sum6/1 -> Scope5/1, R Alpha [rad]/1
  Demux3/1 -> [Rphi_shin]
  Demux3/2 -> [Rgear_shin]
  Demux3/3 -> [Rphi_thigh]
  Demux3/4 -> [Rgear_thigh]
  Demux3/5 -> [Lphi_shin]
  Demux3/6 -> [Lgear_shin]
  Demux3/7 -> [Lphi_thigh]
  Demux3/8 -> [Lgear_thigh]
  Demux3/9 -> [Rphi_Lat]
  Demux3/10 -> [Lphi_Lat]
  Demux3/11 -> [roll]
  Demux3/12 -> [yaw]
  Demux3/13 -> [theta]
  Demux2/13 -> [dtheta]
  Demux2/8 -> [Ldgear_thigh]
  Demux2/10 -> [Ldphi_Lat]
  Demux2/6 -> [Ldgear_shin]
  Demux2/9 -> [Rdphi_Lat]
  Demux2/11 -> [droll]
  Demux2/12 -> [dyaw]
  Demux2/4 -> [Rdgear_thigh]
  Demux2/5 -> [Ldphi_shin]
  Demux2/7 -> [Ldphi_thigh]
  Demux2/1 -> [Rdphi_shin]
  Demux2/3 -> [Rdphi_thigh]
  Demux2/2 -> [Rdgear_shin]
  dq_discrete [rad/2] x13/1 -> Demux2/1
  Trigonometric Function6/1 -> Product4/2
  [roll] -> Trigonometric Function6/1
  Constant6/1 -> Product4/3
  [Lgear_shin] -> Sum11/1
  Sum11/1 -> Gain4/1
  [Lphi_shin] -> Sum11/2
  Gain4/1 -> Scope6/3, L_tau_back_meas [Nm]/1
  [Lgear_thigh] -> Sum10/1
  Sum10/1 -> Gain3/1
  [Lphi_thigh] -> Sum10/2
  Gain3/1 -> Scope6/4, L_tau_front_meas [Nm]/1
  [Rgear_shin] -> Sum13/1
  Sum13/1 -> Gain6/1
  [Rphi_shin] -> Sum13/2
  Gain6/1 -> Scope6/1, R_tau_back_meas [Nm]/1
  [Rgear_thigh] -> Sum12/1
  Sum12/1 -> Gain5/1
  [Rphi_thigh] -> Sum12/2
  Gain5/1 -> Scope6/2, R_tau_front_meas [Nm]/1
  Demux6/1 -> Scope7/1, R Leg Length [m]/1
  Demux7/1 -> Scope7/3, L Leg Length [m]/1
  [Rphi_thigh] -> "R Leg Geometry f(l_seg, l_v, v12_max)"/2(qFront [rad])
  [Rphi_shin] -> "R Leg Geometry f(l_seg, l_v, v12_max)"/1(qBack [rad])
  [Rdphi_shin] -> "R Leg Geometry f(l_seg, l_v, v12_max)"/3(dqBack [rad/s])
  [Rdphi_thigh] -> "R Leg Geometry f(l_seg, l_v, v12_max)"/4(dqFront [rad/s])
  "R Leg Geometry f(l_seg, l_v, v12_max)"/4(virtual hip velocity [rad/s]) -> [Rdphi23]
  "R Leg Geometry f(l_seg, l_v, v12_max)"/2(virtual knee velocity [rad/s]) -> [Rdphi12]
  "R Leg Geometry f(l_seg, l_v, v12_max)"/5(k) -> R Jacobian Constant (k)/1
  [Lphi_thigh] -> "R Leg Geometry f(l_seg, l_v, v12_max)1"/2(qFront [rad])
  [Lphi_shin] -> "R Leg Geometry f(l_seg, l_v, v12_max)1"/1(qBack [rad])
  [Ldphi_shin] -> "R Leg Geometry f(l_seg, l_v, v12_max)1"/3(dqBack [rad/s])
  [Ldphi_thigh] -> "R Leg Geometry f(l_seg, l_v, v12_max)1"/4(dqFront [rad/s])
  "R Leg Geometry f(l_seg, l_v, v12_max)1"/5(k) -> L Jacobian Constant (k)/1
  "R Leg Geometry f(l_seg, l_v, v12_max)"/3(virtual hip angle [rad]) -> R virtual hip angle [rad]/1
  "R Leg Geometry f(l_seg, l_v, v12_max)"/1(virtual knee angle [rad]) -> R virtual knee angle [rad]/1
  "R Leg Geometry f(l_seg, l_v, v12_max)1"/1(virtual knee angle [rad]) -> L virtual knee angle [rad]/1
  "R Leg Geometry f(l_seg, l_v, v12_max)1"/3(virtual hip angle [rad]) -> L virtual hip angle [rad]/1
  "R Leg Geometry f(l_seg, l_v, v12_max)1"/2(virtual knee velocity [rad/s]) -> [Ldphi12]
  "R Leg Geometry f(l_seg, l_v, v12_max)1"/4(virtual hip velocity [rad/s]) -> [Ldphi23]
  Constant11/1 -> Sum18/2
  [Ralpha] -> Mux7/1
  [Lalpha] -> Mux7/2
  Mux7/1 -> Sum18/1
  Sum18/1 -> Demux4/1
  Demux4/1 -> Rgamma [rad]/1
  Demux4/2 -> Lgamma [rad]/1
  [Rdalpha] -> Mux6/1
  [Ldalpha] -> Mux6/2
  Mux6/1 -> Demux1/1
  Demux1/1 -> Rdgamma [rad]/1
  Demux1/2 -> Ldgamma [rad]/1
  q_discrete [rad] x13/1 -> Demux3/1
  RC Demux/1(Out1) -> [qBackR]
  RC Demux/2(Out2) -> [qFrontR]
  RC Demux/3(Out3) -> [qBackL]
  RC Demux/4(Out4) -> [qFrontL]
  RC Demux/5(Out5) -> [qLatR]
  RC Demux/6(Out6) -> [qLatL]
  RC Demux/7(Out7) -> [qBoomRoll]
  RC Demux/8(Out8) -> [qBoomYaw]
  RC Demux/9(Out9) -> [qBoomPitch]
  [q] -> RC Demux/1(In1)
  [dq] -> RC dq demux/1(In1)
  RC dq demux/1(Out1) -> [dqBackR]
  RC dq demux/2(Out2) -> [dqFrontR]
  RC dq demux/3(Out3) -> [dqBackL]
  RC dq demux/4(Out4) -> [dqFrontL]
  RC dq demux/5(Out5) -> [dqLatR]
  RC dq demux/6(Out6) -> [dqLatL]
  RC dq demux/7(Out7) -> [dqBoomRoll]
  RC dq demux/8(Out8) -> [dqBoomYaw]
  RC dq demux/9(Out9) -> [dqBoomPitch]
  L Leg Calculator/4(Leg Width [m]) -> [LLegW]
  Selector26/1 -> Mux8/1
  Selector27/1 -> Mux8/2
  Selector25/1 -> Mux9/2
  Selector24/1 -> Mux9/1
  L Leg Calculator/3(Leg Splay [rad rad/s]) -> Demux8/1, [LLegSplay]
  L Leg Calculator/2(Leg Angle [rad rad/s]) -> [LLegAngle]
  L Leg Calculator/1("Leg Length [m m/s] ") -> [LLegLength]
  Mux8/1 -> L Leg Calculator/2(Back [rad rad/s])
  Mux9/1 -> L Leg Calculator/1(Front [rad rad/s])
  [dqFrontL] -> Selector25/1
  [qFrontL] -> Selector24/1
  [dqBackL] -> Selector27/1
  [qBackL] -> Selector26/1
  R Leg Calculator/4(Leg Width [m]) -> [RLegW]
  Selector16/1 -> Mux4/1
  Selector17/1 -> Mux4/2
  Selector15/1 -> Mux5/2
  Selector14/1 -> Mux5/1
  R Leg Calculator/3(Leg Splay [rad rad/s]) -> Demux9/1, [RLegSplay]
  R Leg Calculator/2(Leg Angle [rad rad/s]) -> [RLegAngle]
  [dqFrontR] -> Selector15/1
  [qFrontR] -> Selector14/1
  [dqBackR] -> Selector17/1
  [qBackR] -> Selector16/1
  R Leg Calculator/1("Leg Length [m m/s] ") -> [RLegLength]
  Mux4/1 -> R Leg Calculator/2(Back [rad rad/s])
  Mux5/1 -> R Leg Calculator/1(Front [rad rad/s])
  [RLegAngle] -> Demux/1
  Demux/1 -> Sum6/2
  [dtheta] -> Sum14/2
  Demux/2 -> Sum14/1
  Sum14/1 -> Scope5/2, R dAlpha [rad/s]/1
  [theta] -> Sum5/3
  Constant12/1 -> Sum5/1
  Sum5/1 -> Scope5/3, L Alpha [rad]/1
  [LLegAngle] -> Demux5/1
  Demux5/1 -> Sum5/2
  [dtheta] -> Sum4/2
  Demux5/2 -> Sum4/1
  Sum4/1 -> Scope5/4, L dAlpha [rad/s]/1
  Demux6/2 -> Scope7/2, R Leg Length Velocity [m/s]/1
  [RLegLength] -> Demux6/1
  Demux7/2 -> Scope7/4, L Leg Length Velocity [m/s]/1
  [LLegLength] -> Demux7/1
  [RLegW] -> Mux33/1
  [LLegW] -> Mux33/2
  [RLegLength] -> Selector31/1
  [LLegLength] -> Selector32/1
  Selector31/1 -> Mux34/1
  Selector32/1 -> Mux34/2
  Selector34/1 -> Mux35/2
  [RLegAngle] -> Selector33/1
  [LLegAngle] -> Selector34/1
  Selector33/1 -> Mux35/1
  [TorsoPitch] -> Selector35/1
  [q] -> Force Estimation/1(q)
  Selector35/1 -> Force Estimation/2(Torso Pitch [rad])
  [RightLeftPrimary] -> Force Estimation/3(Right/Left Primary)
  Force Estimation/3(Left Leg Measured Axial Force [N]) -> Switch1/3, [LLegMeasuredForce]
  Force Estimation/2(Right Leg Measured Axial Force [N]) -> Switch1/1, [RLegMeasuredForce]
  Mux35/1 -> Force Estimation/4(Leg Angle Right/Left [rad rad])
  Mux33/1 -> Force Estimation/5(Leg Width Right/Left [m m])
  Mux34/1 -> Force Estimation/6(Leg Length Right/Left [m m])
  Force Estimation/5("Right [horizontal GRF, vertical GRF] [N N]") -> [RightLegGRFs]
  Force Estimation/6("Left [horizontal GRF, vertical GRF] [N N]") -> [LeftLegGRFs]
  Force Estimation/7(GRFx) -> [GRFx]
  Force Estimation/4(Primary Measured Vertical GRF [N]) -> [PrimaryMeasuredVerticalGRF]
  Force Estimation/1(Vertical GRF [body weight]) -> [GRFy]
  Constant13/1 -> Divide/2
  Selector36/1 -> Divide/1
  [LeftLegGRFs] -> Selector36/1
  Divide/1 -> Scope8/1, L Leg Load [bw]/1
  Constant14/1 -> Divide1/2
  Selector37/1 -> Divide1/1
  [RightLegGRFs] -> Selector37/1
  Divide1/1 -> Scope8/2, R Leg Load [bw]/1
  [Z_dZ] -> Contact State Machine/2("[Z dZ] [m m/s]")
  Contact State Machine/2(Exiting Stance [1/0]) -> Scope3/1, [LeftExitingStance]
  Contact State Machine/1(flight [1/0]) -> [Leftflight]
  [Z_dZ] -> Contact State Machine1/2("[Z dZ] [m m/s]")
  Contact State Machine1/1(flight [1/0]) -> [Rightflight]
  [RLLoad] -> Contact State Machine1/1(Contact Factor [body weight])
  [LLLoad] -> Contact State Machine/1(Contact Factor [body weight])
  Contact State Machine/3(Entering stance [1/0]) -> Scope3/2, [LeftEnteringStance]
  Demux8/1 -> Scope4/1, [Lsplay]
  Demux9/1 -> Scope4/3, [Rsplay]
  Data Type Conversion3/1 -> Goto81/1, R/L Stance/1, R Contact [0/1]/1
  [RightEnteringStance] -> Logical Operator/1
  [LeftEnteringStance] -> Logical Operator/2
  Logical Operator/1 -> Entering stance/1, [EnteringStance]
  [RightEnteringStance] -> S-R Flip-Flop1/1
  [RightExitingStance] -> S-R Flip-Flop1/2
  S-R Flip-Flop1/1 -> Data Type Conversion3/1
  S-R Flip-Flop1/2 -> Terminator1/1
  Data Type Conversion1/1 -> Goto84/1, R/L Stance/2, L Contact [0/1]/1
  [LeftEnteringStance] -> S-R Flip-Flop2/1
  [LeftExitingStance] -> S-R Flip-Flop2/2
  S-R Flip-Flop2/1 -> Data Type Conversion1/1
  S-R Flip-Flop2/2 -> Terminator2/1
  [yaw] -> Gain1/1
  Trigonometric Function4/1 -> Product5/2
  [roll] -> Trigonometric Function4/1
  Constant7/1 -> Product5/3
  Product5/1 -> Sum7/2, Scope/2, [xTorso]
  Integrator/1 -> Sum7/1, Scope/1
  Sum7/1 -> Scope/3
  Contact State Machine1/2(Exiting Stance [1/0]) -> Scope2/1, [RightExitingStance]
  Contact State Machine1/3(Entering stance [1/0]) -> Scope2/2, [RightEnteringStance]
  Demux8/2 -> Scope4/2
  Demux9/2 -> Scope4/4
  [RightLeftPrimary] -> Switch1/2
  Switch1/1 -> [PrimaryAxialLegForce]
  Gain/1 -> Product4/1
  Gain1/1 -> Product5/1

== system atrias_gear_dynamics/control/Virtual Neuromuscular Control ==
  note: High-Level
      | Control
  note: Neural
      | Control
  note: Muscle
      | Dynamics
  note: Jacobian Mapping
  Constant10 : Constant  Value=nmc_TrCtrlPar
  Constant12 : Constant  Value=nmc_BLCtrlPar
  Constant2 : Constant  Value=nmc_LLCtrlPar
  Constant5 : Constant  Value=nmc_StCtrlPar
  Constant6 : Constant  Value=nmc_FPCtrlPar
  Constant9 : Constant  Value=nmc_SwCtrlPar
  Higher Control Layer : Subsystem
  Muscle Layer : Subsystem
  Neural Control Layer : Subsystem
  Torque Distribution : Subsystem
  RtauB_des [Nm] : Outport
  RtauF_des [Nm] : Outport  Port=2
  LtauB_des [Nm] : Outport  Port=3
  LtauF_des [Nm] : Outport  Port=4
  tag scope: FPCtrlPar=global, Jinv_trans_L=global, Jinv_trans_R=global, LLCtrlPar=global, StCtrlPar=global, SwCtrlPar=global, TrCtrlPar=global, theta0=global
  wires:
  Torque Distribution/6(L J_inv_transpose [2x2]) -> [Jinv_trans_L]
  Torque Distribution/5(L tauF [Nm]) -> LtauF_des [Nm]/1
  Torque Distribution/4(L tauB [Nm]) -> LtauB_des [Nm]/1
  Torque Distribution/3(R J_inv_transpose [2x2]) -> [Jinv_trans_R]
  [LM12] -> Torque Distribution/4(L tauK_des [Nm])
  [LM23] -> Torque Distribution/5(L tauH_des [Nm])
  [k_R] -> Torque Distribution/3(R Jacobian Constant (k))
  [k_L] -> Torque Distribution/6(L Jacobian Constant (k))
  Torque Distribution/1(R tauB [Nm]) -> RtauB_des [Nm]/1
  Torque Distribution/2(R tauF [Nm]) -> RtauF_des [Nm]/1
  [RM23] -> Torque Distribution/2(R tauH_des [Nm])
  [RM12] -> Torque Distribution/1(R tauK_des [Nm])
  Constant6/1 -> [FPCtrlPar]
  Constant10/1 -> [TrCtrlPar]
  Constant9/1 -> [SwCtrlPar]
  Constant2/1 -> [LLCtrlPar]
  Constant5/1 -> [StCtrlPar]
  Constant12/1 -> [theta0]

== system atrias_gear_dynamics/control/switch Ctrl ==
  VNMC : Inport
  RC : Inport  Port=2
  Constant : Constant  Value=0
  Demux1 : Demux  Outputs=2
  Demux2 : Demux  Outputs=2
  Mux7 : Mux  Inputs=2
  Scope : Scope  Commented=on  NumInputPorts=5
  Scope1 : Scope  NumInputPorts=5
  Switch{1..4} (4 alike) : Switch  Criteria=u2 > Threshold  Threshold=.5
  selected : Outport
  wires:
  Switch2/1 -> Scope/4, selected/1
  Switch1/1 -> Switch2/1
  Constant/1 -> Switch1/2
  [RFootCnt] -> Scope1/1, Switch3/2
  VNMC/1 -> Demux1/1, [vnmc_trq]
  RC/1 -> Demux2/1, [rc_trq]
  Demux1/1 -> Scope1/3, Switch3/1
  Demux2/1 -> Scope1/5, Switch3/3
  [LFootCnt] -> Scope1/2, Switch4/2
  Demux1/2 -> Switch4/1
  Demux2/2 -> Switch4/3
  Switch3/1 -> Scope1/4, Mux7/1
  Switch4/1 -> Mux7/2
  Mux7/1 -> [hybrid_trq]
  [rc_trq] -> Scope/3, Switch2/3
  [vnmc_on] -> Scope/5, Switch2/2
  [vnmc_trq] -> Scope/1, Switch1/3
  [hybrid_trq] -> Scope/2, Switch1/1

== system atrias_gear_dynamics/ATRIAS_sim/Discrete Derivative/discrete difference ==
  note: q Order:
      |
      | backJointR
      | backGearR
      | frontJointR
      | frontGearR
      |
      | backJointL
      | backGearL
      | frontJointL
      | frontGearL
      |
      | latR
      | latL
      |
      | boomRoll
      | boomYaw
      | boomPitch
  in : Inport
  Demux : Demux  Outputs=13
  Mux : Mux  Inputs=13
  difference : simulink/Discrete/Difference  ICPrevInput=sm.shin_initial_r  InputProcessing=Columns as channels (frame based)  OutMin=[]  OutMax=[]  OutDataType=fixdt(1, 16)  OutScaling=2^-10  DoSatur=off
  difference1 : simulink/Discrete/Difference  ICPrevInput=sm.shin_initial_r  InputProcessing=Columns as channels (frame based)  OutMin=[]  OutMax=[]  OutDataType=fixdt(1, 16)  OutScaling=2^-10  DoSatur=off
  difference10 : simulink/Discrete/Difference  ICPrevInput=sm.initial_boom_roll  InputProcessing=Columns as channels (frame based)  OutMin=[]  OutMax=[]  OutDataType=fixdt(1, 16)  OutScaling=2^-10  DoSatur=off
  difference11 : simulink/Discrete/Difference  ICPrevInput=sm.initial_boom_yaw  InputProcessing=Columns as channels (frame based)  OutMin=[]  OutMax=[]  OutDataType=fixdt(1, 16)  OutScaling=2^-10  DoSatur=off
  difference12 : simulink/Discrete/Difference  ICPrevInput=sm.initial_boom_pitch  InputProcessing=Columns as channels (frame based)  OutMin=[]  OutMax=[]  OutDataType=fixdt(1, 16)  OutScaling=2^-10  DoSatur=off
  difference2 : simulink/Discrete/Difference  ICPrevInput=sm.thigh_initial_r  InputProcessing=Columns as channels (frame based)  OutMin=[]  OutMax=[]  OutDataType=fixdt(1, 16)  OutScaling=2^-10  DoSatur=off
  difference3 : simulink/Discrete/Difference  ICPrevInput=sm.thigh_initial_r  InputProcessing=Columns as channels (frame based)  OutMin=[]  OutMax=[]  OutDataType=fixdt(1, 16)  OutScaling=2^-10  DoSatur=off
  difference4 : simulink/Discrete/Difference  ICPrevInput=sm.shin_initial_l  InputProcessing=Columns as channels (frame based)  OutMin=[]  OutMax=[]  OutDataType=fixdt(1, 16)  OutScaling=2^-10  DoSatur=off
  difference5 : simulink/Discrete/Difference  ICPrevInput=sm.shin_initial_l  InputProcessing=Columns as channels (frame based)  OutMin=[]  OutMax=[]  OutDataType=fixdt(1, 16)  OutScaling=2^-10  DoSatur=off
  difference6 : simulink/Discrete/Difference  ICPrevInput=sm.thigh_initial_l  InputProcessing=Columns as channels (frame based)  OutMin=[]  OutMax=[]  OutDataType=fixdt(1, 16)  OutScaling=2^-10  DoSatur=off
  difference7 : simulink/Discrete/Difference  ICPrevInput=sm.thigh_initial_l  InputProcessing=Columns as channels (frame based)  OutMin=[]  OutMax=[]  OutDataType=fixdt(1, 16)  OutScaling=2^-10  DoSatur=off
  difference8 : simulink/Discrete/Difference  ICPrevInput=sm.initial_hip_roll  InputProcessing=Columns as channels (frame based)  OutMin=[]  OutMax=[]  OutDataType=fixdt(1, 16)  OutScaling=2^-10  DoSatur=off
  difference9 : simulink/Discrete/Difference  ICPrevInput=sm.initial_hip_roll  InputProcessing=Columns as channels (frame based)  OutMin=[]  OutMax=[]  OutDataType=fixdt(1, 16)  OutScaling=2^-10  DoSatur=off
  out : Outport
  wires:
  Demux/1 -> difference/1
  in/1 -> Demux/1
  Mux/1 -> out/1
  Demux/2 -> difference1/1
  difference1/1 -> Mux/2
  Demux/3 -> difference2/1
  difference2/1 -> Mux/3
  Demux/4 -> difference3/1
  difference3/1 -> Mux/4
  Demux/5 -> difference4/1
  difference4/1 -> Mux/5
  Demux/6 -> difference5/1
  difference5/1 -> Mux/6
  Demux/7 -> difference6/1
  difference6/1 -> Mux/7
  Demux/8 -> difference7/1
  difference7/1 -> Mux/8
  Demux/9 -> difference8/1
  difference8/1 -> Mux/9
  Demux/10 -> difference9/1
  difference9/1 -> Mux/10
  Demux/11 -> difference10/1
  difference10/1 -> Mux/11
  Demux/12 -> difference11/1
  difference11/1 -> Mux/12
  Demux/13 -> difference12/1
  difference12/1 -> Mux/13
  difference/1 -> Mux/1

== system atrias_gear_dynamics/ATRIAS_sim/Mechanical System Layer/Boom ==
  CS1 to CS2 : sm_lib/Frames and Transforms/Rigid Transform  TranslationMethod=Cartesian  TranslationStandardOffset=0  TranslationLengthUnit=m  TranslationStandardAxis=+Z  TranslationCartesianOffset=sm.boom_12  TranslationROffset=0  TranslationROffsetUnits=m  TranslationZOffset=0  TranslationZOffsetUnits=m  TranslationThetaOffset=0  TranslationThetaOffsetUnits=deg  RotationMethod=None  RotationAngleUnits=deg  RotationStandardAxis=+Z  RotationAngle=0  RotationArbitraryAxis=[0 0 1]  FollAlignAxisA=+X  BaseAlignAxisA=+Y  FollAlignAxisB=+Y  BaseAlignAxisB=+Z  RotationSequenceAxes=FollowerAxes  RotationSequence=XYX  RotationSequenceAngles=[0 0 0]  RotationSequenceAnglesUnits=deg  RotationMatrix=[1 0 0; 0 1 0; 0 0 1]
  Frame Data : Subsystem
  Solid : sm_lib/Body Elements/Solid  InertiaType=Custom  Mass=sm.m_boom  MassUnits=kg  CenterOfMass=sm.com_boom  CenterOfMassUnits=m  MomentsOfInertia=sm.i_boom_moments  MomentsOfInertiaUnits=kg*m^2  ProductsOfInertia=sm.i_boom_products  ProductsOfInertiaUnits=kg*m^2  DensityBased=on  Density=1000  DensityUnits=kg/(m^3)  DoExposeReferenceFrame=on  SerializedFrames=<Frames/>  GraphicType=FromGeometry  MarkerShape=Sphere  MarkerSize=10  MarkerSizeUnits=m  GraphicVisPropType=AdvancedVisualProperties  GraphicDiffuseColor=sm.boom_color_d  GraphicSpecularColor=[0.5 0.5 0.5 1.0]  GraphicAmbientColor=[sm.boom_color_d*0.5 1.0]  GraphicEmissiveColor=[0.0 0.0 0.0 1.0]  GraphicShininess=128  GraphicOpacity=1.0  GeometryShape=FromFile  RectangleSize=[1 1]  RectangleSizeUnits=m  BrickDimensions=[1 1 1]  BrickDimensionUnits=m  CylinderRadius=1  CylinderRadiusUnits=m  CylinderLength=1  CylinderLengthUnits=m  SphereRadius=1  SphereRadiusUnits=m  EllipsoidRadii=[1 1 1]  EllipsoidRadiiUnits=m  ExtrusionCrossSection=[1 1; -1 1; -1 -1; 1 -1]  ExtrusionCrossSectionUnits=m  ExtrusionLength=1  ExtrusionLengthUnits=m  PolygonNumSides=3  PolygonOuterRadius=1  PolygonOuterRadiusUnits=m  ExtGeomFileType=STL  ExtGeomFileName=../models/boom_roll.stl  ExtGeomFileUnits=m  RevolutionCrossSection=[1 1; 1 -1; 2 -1; 2 1]  RevolutionCrossSectionUnits=m  RevolutionExtent=Full  RevolutionAngle=180  RevolutionAngleUnits=deg
  CS1 : PMIOPort  Port=1  Side=Left
  CS2 : PMIOPort  Port=2  Side=Right
  connections:
  CS1/RConn1 -- Frame Data/LConn1 -- CS1 to CS2/LConn1 -- Solid/RConn1
  CS2/RConn1 -- CS1 to CS2/RConn1
